simulink model "SWC_TRSP"  (R2020a)
settings: Solver=FixedStepDiscrete  StartTime=0.0  StopTime=0.15  FixedStep=0.0001  RelTol=1e-3
values from neighbouring files (symbols this model uses):
  CAL_TRSP_18VHSVoltCountTrh_s16 = 0.0    [SWC_TRSP_DataDictionary.sldd]
  CAL_TRSP_18VHSVoltDebTrh_s16 = 0.0    [SWC_TRSP_DataDictionary.sldd]
  CAL_TRSP_18VHSVoltErrRst_b = 0.0    [SWC_TRSP_DataDictionary.sldd]
  CAL_TRSP_18VHSVoltHiLim_u16 = 0.0    [SWC_TRSP_DataDictionary.sldd]
  CAL_TRSP_18VHSVoltLoLim_u16 = 0.0    [SWC_TRSP_DataDictionary.sldd]
  CAL_TRSP_1V8CPLDVoltCountTrh_s16 = 0.0    [SWC_TRSP_DataDictionary.sldd]
  CAL_TRSP_1V8CPLDVoltDebTrh_s16 = 0.0    [SWC_TRSP_DataDictionary.sldd]
  CAL_TRSP_1V8CPLDVoltErrRst_b = 0.0    [SWC_TRSP_DataDictionary.sldd]
  CAL_TRSP_1V8CPLDVoltHiLim_u16 = 0.0    [SWC_TRSP_DataDictionary.sldd]
  CAL_TRSP_1V8CPLDVoltLoLim_u16 = 0.0    [SWC_TRSP_DataDictionary.sldd]
  CAL_TRSP_3V3CPLDVoltCountTrh_s16 = 0.0    [SWC_TRSP_DataDictionary.sldd]
  CAL_TRSP_3V3CPLDVoltDebTrh_s16 = 0.0    [SWC_TRSP_DataDictionary.sldd]
  CAL_TRSP_3V3CPLDVoltErrRst_b = 0.0    [SWC_TRSP_DataDictionary.sldd]
  CAL_TRSP_3V3CPLDVoltHiLim_u16 = 0.0    [SWC_TRSP_DataDictionary.sldd]
  CAL_TRSP_3V3CPLDVoltLoLim_u16 = 0.0    [SWC_TRSP_DataDictionary.sldd]
  CAL_TRSP_AgTimecompCtl_u8 = 0.0    [SWC_TRSP_DataDictionary.sldd]
  CAL_TRSP_CurrRngCountTrh_s16 = 0.0    [SWC_TRSP_DataDictionary.sldd]
  CAL_TRSP_CurrRngDebTrh_s16 = 0.0    [SWC_TRSP_DataDictionary.sldd]
  CAL_TRSP_CurrRngErrRst_b = 0.0    [SWC_TRSP_DataDictionary.sldd]
  CAL_TRSP_CurrSumCountTrh_s16 = 0.0    [SWC_TRSP_DataDictionary.sldd]
  CAL_TRSP_CurrSumDebTrh_s16 = 0.0    [SWC_TRSP_DataDictionary.sldd]
  CAL_TRSP_CurrSumErrRst_b = 0.0    [SWC_TRSP_DataDictionary.sldd]
  CAL_TRSP_CurrSumLim_f32 = 0.0    [SWC_TRSP_DataDictionary.sldd]
  CAL_TRSP_Diff_UBR_SBCLim_f32 = 0.0    [SWC_TRSP_DataDictionary.sldd]
  CAL_TRSP_flgChangPha_b = 0.0    [SWC_TRSP_DataDictionary.sldd]
  CAL_TRSP_iPhasSensVoltCountTrh_s16 = 0.0    [SWC_TRSP_DataDictionary.sldd]
  CAL_TRSP_iPhasSensVoltDebTrh_s16 = 0.0    [SWC_TRSP_DataDictionary.sldd]
  CAL_TRSP_iPhasSensVoltErrRst_b = 0.0    [SWC_TRSP_DataDictionary.sldd]
  CAL_TRSP_iPhasSensVoltHiLim_u16 = 0.0    [SWC_TRSP_DataDictionary.sldd]
  CAL_TRSP_iPhasSensVoltLoLim_u16 = 0.0    [SWC_TRSP_DataDictionary.sldd]
  CAL_TRSP_iPhaUOffset_f32 = 0.0    [SWC_TRSP_DataDictionary.sldd]
  CAL_TRSP_iPhaVOffset_f32 = 0.0    [SWC_TRSP_DataDictionary.sldd]
  CAL_TRSP_iPhaWOffset_f32 = 0.0    [SWC_TRSP_DataDictionary.sldd]
  CAL_TRSP_iUCnvFac_f32 = 0.0    [SWC_TRSP_DataDictionary.sldd]
  CAL_TRSP_iVCnvFac_f32 = 0.0    [SWC_TRSP_DataDictionary.sldd]
  CAL_TRSP_iWCnvFac_f32 = 0.0    [SWC_TRSP_DataDictionary.sldd]
  CAL_TRSP_OfstErrRst_b = 0.0    [SWC_TRSP_DataDictionary.sldd]
  CAL_TRSP_OfstRngHiLim_f32 = 0.0    [SWC_TRSP_DataDictionary.sldd]
  CAL_TRSP_OfstRngLoLim_f32 = 0.0    [SWC_TRSP_DataDictionary.sldd]
  CAL_TRSP_ReqTrqCountTrh_s16 = 0.0    [SWC_TRSP_DataDictionary.sldd]
  CAL_TRSP_ReqTrqDebTrh_s16 = 0.0    [SWC_TRSP_DataDictionary.sldd]
  CAL_TRSP_ReqTrqErrRst_b = 0.0    [SWC_TRSP_DataDictionary.sldd]
  CAL_TRSP_ReqTrqHiLim_f32 = 0.0    [SWC_TRSP_DataDictionary.sldd]
  CAL_TRSP_ReqTrqLoLim_f32 = 0.0    [SWC_TRSP_DataDictionary.sldd]
  CAL_TRSP_RslvExciCountTrh_s16 = 0.0    [SWC_TRSP_DataDictionary.sldd]
  CAL_TRSP_RslvExciDebTrh_s16 = 0.0    [SWC_TRSP_DataDictionary.sldd]
  CAL_TRSP_RslvExciErrRst_b = 0.0    [SWC_TRSP_DataDictionary.sldd]
  CAL_TRSP_RslvMaxSele_u8 = 0.0    [SWC_TRSP_DataDictionary.sldd]
  CAL_TRSP_RslvMinSele_u8 = 0.0    [SWC_TRSP_DataDictionary.sldd]
  CAL_TRSP_RslvRngCosNHiLim_u16 = 0.0    [SWC_TRSP_DataDictionary.sldd]
  CAL_TRSP_RslvRngCosNLoLim_u16 = 0.0    [SWC_TRSP_DataDictionary.sldd]
  CAL_TRSP_RslvRngCosPHiLim_u16 = 0.0    [SWC_TRSP_DataDictionary.sldd]
  CAL_TRSP_RslvRngCosPLoLim_u16 = 0.0    [SWC_TRSP_DataDictionary.sldd]
  CAL_TRSP_RslvRngCountTrh_s16 = 0.0    [SWC_TRSP_DataDictionary.sldd]
  CAL_TRSP_RslvRngDebTrh_s16 = 0.0    [SWC_TRSP_DataDictionary.sldd]
  CAL_TRSP_RslvRngErrRst_b = 0.0    [SWC_TRSP_DataDictionary.sldd]
  CAL_TRSP_RslvRngExciHiLim_u16 = 0.0    [SWC_TRSP_DataDictionary.sldd]
  CAL_TRSP_RslvRngExciLoLim_u16 = 0.0    [SWC_TRSP_DataDictionary.sldd]
  CAL_TRSP_RslvRngSinNHiLim_u16 = 0.0    [SWC_TRSP_DataDictionary.sldd]
  CAL_TRSP_RslvRngSinNLoLim_u16 = 0.0    [SWC_TRSP_DataDictionary.sldd]
  CAL_TRSP_RslvRngSinPHiLim_u16 = 0.0    [SWC_TRSP_DataDictionary.sldd]
  CAL_TRSP_RslvRngSinPLoLim_u16 = 0.0    [SWC_TRSP_DataDictionary.sldd]
  CAL_TRSP_RslvSensVoltCountTrh_s16 = 0.0    [SWC_TRSP_DataDictionary.sldd]
  CAL_TRSP_RslvSensVoltDebTrh_s16 = 0.0    [SWC_TRSP_DataDictionary.sldd]
  CAL_TRSP_RslvSensVoltErrRst_b = 0.0    [SWC_TRSP_DataDictionary.sldd]
  CAL_TRSP_RslvSensVoltHiLim_u16 = 0.0    [SWC_TRSP_DataDictionary.sldd]
  CAL_TRSP_RslvSensVoltLoLim_u16 = 0.0    [SWC_TRSP_DataDictionary.sldd]
  CAL_TRSP_RslvSqrtCountTrh_s16 = 0.0    [SWC_TRSP_DataDictionary.sldd]
  CAL_TRSP_RslvSqrtDebTrh_s16 = 0.0    [SWC_TRSP_DataDictionary.sldd]
  CAL_TRSP_RslvSqrtErrRst_b = 0.0    [SWC_TRSP_DataDictionary.sldd]
  CAL_TRSP_RslvSqrtHiLim_u16 = 0.0    [SWC_TRSP_DataDictionary.sldd]
  CAL_TRSP_RslvSqrtLoLim_u16 = 0.0    [SWC_TRSP_DataDictionary.sldd]
  CAL_TRSP_SpeedCtlMode_u8 = 0.0    [SWC_TRSP_DataDictionary.sldd]
  CAL_TRSP_TorqueCtlMode_u8 = 0.0    [SWC_TRSP_DataDictionary.sldd]
  CAL_TRSP_UB_SBCCnvFac_f32 = 0.0    [SWC_TRSP_DataDictionary.sldd]
  CAL_TRSP_UBRVoltCountTrh_s16 = 0.0    [SWC_TRSP_DataDictionary.sldd]
  CAL_TRSP_UBRVoltDebTrh_s16 = 0.0    [SWC_TRSP_DataDictionary.sldd]
  CAL_TRSP_UBRVoltErrRst_b = 0.0    [SWC_TRSP_DataDictionary.sldd]
  CAL_TRSP_UBRWIDECnvFac_f32 = 0.0    [SWC_TRSP_DataDictionary.sldd]
  CAL_TRSP_UCurrRngHiLim_f32 = 0.0    [SWC_TRSP_DataDictionary.sldd]
  CAL_TRSP_UCurrRngLoLim_f32 = 0.0    [SWC_TRSP_DataDictionary.sldd]
  CAL_TRSP_VCurrRngHiLim_f32 = 0.0    [SWC_TRSP_DataDictionary.sldd]
  CAL_TRSP_VCurrRngLoLim_f32 = 0.0    [SWC_TRSP_DataDictionary.sldd]
  CAL_TRSP_WCurrRngHiLim_f32 = 0.0    [SWC_TRSP_DataDictionary.sldd]
  CAL_TRSP_WCurrRngLoLim_f32 = 0.0    [SWC_TRSP_DataDictionary.sldd]
  GLB_TRSP_CircAge_f32 = 0.0    [SWC_TRSP_DataDictionary.sldd]
  GLB_TRSP_MotorPole_u8 = 0.0    [SWC_TRSP_DataDictionary.sldd]
  GLB_TRSP_Sixty_f32 = 0.0    [SWC_TRSP_DataDictionary.sldd]
libraries: simulink x22
(part 13 of 13)

== system SWC_TRSP/SWC_TRSP_10ms_sys/CANSigChk/Debouncer15/Count ==
  CountTrh : Inport
  Enable : EnablePort
  Add : Sum
  Constant : Constant  OutDataTypeStr=int16
  Constant1 : Constant  Value=0  OutDataTypeStr=int16
  Delay : Delay  DelayLength=1
  Relational Operator : RelationalOperator  OutDataTypeStr=boolean  RndMeth=Simplest
  Switch : Switch  Criteria=u2 > Threshold
  Count : Outport
  wires:
  Switch/1 -> Delay/1, Count/1
  Constant/1 -> Add/1
  Relational Operator/1 -> Switch/2
  Add/1 -> Relational Operator/1, Switch/3
  Constant1/1 -> Switch/1
  CountTrh/1 -> Relational Operator/2
  Delay/1 -> Add/2

== system SWC_TRSP/SWC_TRSP_1ms_sys/OfstAgChk/OfstChk/Lock ==
  BooleanIN : Inport
  Rst : Inport  Port=2
  Boolean_ZERO : Constant  Value=0  OutDataTypeStr=boolean
  Logical Operator : Logic  Operator=OR  AllPortsSameDT=off  OutDataTypeStr=boolean
  Switch1 : Switch  Criteria=u2 ~= 0
  Unit Delay1 : UnitDelay  SampleTime=-1  HasFrameUpgradeWarning=on
  OutLock : Outport  VectorParamsAs1DForOutWhenUnconnected=off
  wires:
  Logical Operator/1 -> Unit Delay1/1, OutLock/1
  Unit Delay1/1 -> Switch1/3
  Boolean_ZERO/1 -> Switch1/1
  Rst/1 -> Switch1/2
  Switch1/1 -> Logical Operator/2
  BooleanIN/1 -> Logical Operator/1

== system SWC_TRSP/SWC_TRSP_1ms_sys/OfstAgChk/OfstChk/OfstRngChk ==
  TRSP_OfstRngChkVal : Inport
  TRSP_HiTrh : Inport  Port=2
  TRSP_LoTrh : Inport  Port=3
  Logical Operator : Logic  Operator=OR  AllPortsSameDT=off  OutDataTypeStr=boolean
  Relational Operator : RelationalOperator  Operator=<  OutDataTypeStr=boolean  RndMeth=Simplest
  Relational Operator1 : RelationalOperator  Operator=>  OutDataTypeStr=boolean  RndMeth=Simplest
  TRSP_OfstRngChkRslt : Outport
  wires:
  Relational Operator1/1 -> Logical Operator/1
  TRSP_LoTrh/1 -> Relational Operator/2
  TRSP_OfstRngChkVal/1 -> Relational Operator1/1, Relational Operator/1
  Logical Operator/1 -> TRSP_OfstRngChkRslt/1
  TRSP_HiTrh/1 -> Relational Operator1/2
  Relational Operator/1 -> Logical Operator/2
